simulink model "pmsm_drive_st"  (R2014a)
settings: Solver=ode3  SolverMode=SingleTasking  StartTime=0.0  StopTime=1  FixedStep=Ts  RelTol=1e-4
PreLoadFcn:
  | Ts=1e-5;
InitFcn:
  | Ts=1e-5;
StartFcn:
  | tic;
StopFcn:
  | toc;
undefined symbols (not defined in the file or in its folder): Acid, DiscIntNeverNeededParam, Lead
libraries: powerlib x10, electricdrivelib x1
Description:
  | Copyright 2008 The MathWorks(TM), Inc.
settings Model: ExtModeTrigMode=oneshot  ExtModeArmWhenConnect=off  ExtModeAutoUpdateStatusClock=off  Creator=patrice  LastModifiedBy=cosorio
settings DataIOCC: ExternalInput=[]  LimitDataPoints=off  SignalLoggingSaveFormat=ModelDataLogs  SaveOutput=off  SaveTime=off  SignalLoggingName=sigsOut
settings OptimizationCC: BlockReduction=off  BooleanDataType=off  ExpressionDepthLimit=2147483647  InitFltsAndDblsToZero=on  EfficientMapNaN2IntZero=off  OptimizeModelRefInitCode=on  LifeSpan=1
settings DebuggingCC: UnderspecifiedInitializationDetection=Classic  CheckExecutionContextPreStartOutputMsg=on  CheckExecutionContextRuntimeOutputMsg=on  SignalResolutionControl=TryResolveAllWithWarning  SolverPrmCheckMsg=none  MultiTaskDSMMsg=warning  MultiTaskCondExecSysMsg=none  SigSpecEnsureSampleTimeMsg=none  FcnCallInpInsideContextMsg=UseLocalSettings  StateNameClashWarn=warning
settings HardwareCC: TargetLongLongMode=on  TargetIntDivRoundTo=Zero  TargetEndianess=LittleEndian  TargetHWDeviceType=MATLAB Host  ProdEqTarget=off
settings RTWCC: SystemTargetFile=ert.tlc  TemplateMakefile=ert_default_tmf  Description=Embedded Coder  GenerateReport=on  ProcessScript=ert_make_rtw_hook  IncludeHyperlinkInReport=on  LaunchReport=on  IncludeERTFirstTime=on  GenerateTraceInfo=on  GenerateTraceReport=on  GenerateTraceReportSl=on  GenerateTraceReportSf=on  GenerateTraceReportEml=on  GenerateWebview=on  GenerateCodeMetricsReport=on
settings CodeAppCC: IgnoreCustomStorageClasses=off
settings ERTTargetCC: ParMdlRefBuildCompliant=on  CompOptLevelCompliant=on  ConcurrentExecutionCompliant=on  ERTFirstTimeCompliant=on  ModelStepFunctionPrototypeControlCompliant=on  CPPClassGenCompliant=on  InlinedParameterPlacement=Hierarchical  ERTCustomFileTemplate=example_file_process.tlc
settings SimscapeCC: ExplicitSolverDiagnosticOptions=none

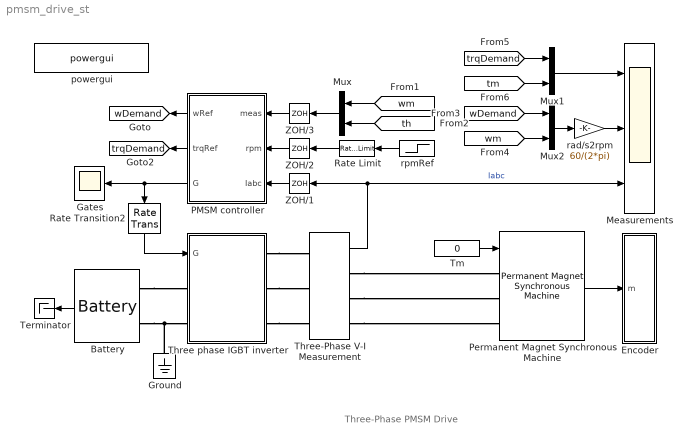
== system pmsm_drive_st ==
  note: Three-Phase PMSM Drive
  Battery : electricdrivelib/Extra Sources/Battery  BatType=Lead-Acid  ShowDetailedParameters=off  NomV=500  NomQ=1200  SOC=80  PresetModel=off  MaxQ=1250  FullV=517  Dis_rate=240  R=0.0041667  Normal_OP=372.3333  expZone="[512           4]"  Dis_Char=off  current=[10 30]  Units=Ampere-hour  Batt_Tr=1
  Encoder : Subsystem
  Gates : Scope
      settings: YMin=-0.2  YMax=1.2  MaxDataPoints=50000
  Ground : powerlib/Elements/Ground  LConnTagsString=a
  Measurements : Scope  NumInputPorts=3
      settings: YMin=-100~0~-2200  YMax=600~250~2200  SaveName=ScopeData4  MaxDataPoints=50000
  Mux : Mux  Inputs=2
  Mux1 : Mux  Inputs=2
  Mux2 : Mux  Inputs=2
  PMSM controller : Subsystem  TreatAsAtomicUnit=on  SystemSampleTime=1e-4
  Permanent Magnet Synchronous Machine : powerlib/Machines/Permanent Magnet Synchronous Machine  NbPhases=3  FluxDistribution=Sinusoidal  RotorType=Salient-pole  MechanicalLoad=Torque Tm  PresetModel=No  ShowDetailedParameters=on  MeasurementBus=off  Resistance=0.013  Inductance=8.5e-3  dqInductances=[0.0002, 0.0001995]  La=0.000835  MachineConstant=Flux linkage established by magnets (V.s)  Flux=0.03  VoltageCst=32.6484  TorqueCst=0.27  Flat=0  Mechanical=[10, 0, 6]  PolePairs=4  InitialConditions=[0,0, 166,-166]  InitialConditions5ph=[0 0 0 0 0 0]  TsPowergui=0  TsBlock=-1  RefAngle=90 degrees behind phase A axis (modified Park)
      settings: AttributesFormatString=\n
  Rate Limit : RateLimiter  RisingSlewLimit=400  FallingSlewLimit=-400  SampleTimeMode=inherited
  Rate Transition2 : RateTransition
  Terminator : Terminator
  Three phase IGBT inverter : Subsystem
  Three-Phase V-I Measurement : powerlib/Measurements/Three-Phase V-I Measurement  VoltageMeasurement=no  SetLabelV=off  LabelV=Vabc  Vpu=off  VpuLL=off  CurrentMeasurement=yes  SetLabelI=off  LabelI=Iabc  Ipu=off  Pbase=100e6  Vbase=500e3  OutputType=Complex  PhasorSimulation=off  PSBequivalent=0
  Tm : Constant  Value=0  SampleTime=Ts
  ZOH/1 : ZeroOrderHold  SampleTime=1e-4
  ZOH/2 : ZeroOrderHold  SampleTime=1e-4
  ZOH/3 : ZeroOrderHold  SampleTime=1e-4
  powergui : powerlib/powergui  SimulationMode=Discrete  SolverType=Tustin  SampleTime=Ts  frequency=60  SPID=off  DisableSnubberDevices=off  DisableRonSwitches=off  DisableVfSwitches=off  SwTol=0  Interpol=off  DisplayEquations=off  Ts=0  methode=off  frequencyindice=0  Pbase=100e6  ErrMax=1e-4  Iterations=50  UnitsV=kV  UnitsW=MW  FunctionMessages=off  echomessages=off  HookPort=off  EnableUseOfTLC=off  x0status=blocks  RestoreLinks=warning  ResistiveCurrentMeasurement=off  Frange=[0:2:500]  Ylog=off  Xlog=on  ShowGrid=off  save=off  variable=ZData  structure=Vmod  ZoomFFT=on  StartTime=2.4  cycles=10  DisplayStyle=1  fundamental=100  FreqAxis=on  MaxFrequency=6500  frequencyindicesteady=1  RmsSteady=1  display=off
  rad/s2rpm : Gain  Gain=60/(2*pi)
  rpmRef : Step  Time=0.1  After=200  SampleTime=1e-4
  tag scope: trqDemand=global, wDemand=global
  wires:
  rpmRef/1 -> Rate Limit/1
  ZOH/1/1 -> PMSM controller/3(Iabc)
  ZOH/2/1 -> PMSM controller/2(rpm)
  ZOH/3/1 -> PMSM controller/1(meas)
  [th] -> Mux/2
  [wm] -> Mux/1
  Mux/1 -> ZOH/3/1
  rad/s2rpm/1 -> Measurements/2
  Mux2/1 -> rad/s2rpm/1
  [wm] -> Mux2/2
  [wDemand] -> Mux2/1
  Mux1/1 -> Measurements/1
  [tm] -> Mux1/2
  [trqDemand] -> Mux1/1
  Battery/1 -> Terminator/1
  PMSM controller/3(G) -> Rate Transition2/1, Gates/1
  Rate Transition2/1 -> Three phase IGBT inverter/1(G)
  Permanent Magnet Synchronous Machine/1 -> Encoder/1(m)
  Tm/1 -> Permanent Magnet Synchronous Machine/1
  Rate Limit/1 -> ZOH/2/1
  Three-Phase V-I Measurement/1 -> Measurements/3, ZOH/1/1  "Iabc"
  PMSM controller/1(wRef) -> [wDemand]
  PMSM controller/2(trqRef) -> [trqDemand]
  connections:
  Battery/LConn2 -- Ground/LConn1 -- Three phase IGBT inverter/LConn2
  Battery/LConn1 -- Three phase IGBT inverter/LConn1
  Three-Phase V-I Measurement/RConn1 -- Permanent Magnet Synchronous Machine/LConn1
  Three-Phase V-I Measurement/RConn2 -- Permanent Magnet Synchronous Machine/LConn2
  Three-Phase V-I Measurement/RConn3 -- Permanent Magnet Synchronous Machine/LConn3
  Three phase IGBT inverter/RConn1 -- Three-Phase V-I Measurement/LConn1
  Three phase IGBT inverter/RConn2 -- Three-Phase V-I Measurement/LConn2
  Three phase IGBT inverter/RConn3 -- Three-Phase V-I Measurement/LConn3

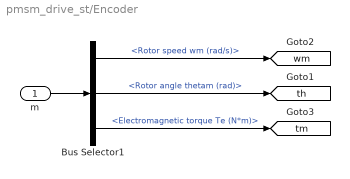
== system pmsm_drive_st/Encoder ==
  m : Inport
  Bus Selector1 : BusSelector  OutputSignals=Rotor speed wm (rad/s),Rotor angle thetam (rad),Electromagnetic torque Te (N*m)
  tag scope: th=global, tm=global, wm=global
  wires:
  Bus Selector1/1 -> [wm]  "<Rotor speed wm (rad/s)>"
  Bus Selector1/3 -> [tm]  "<Electromagnetic torque Te (N*m)>"
  m/1 -> Bus Selector1/1
  Bus Selector1/2 -> [th]  "<Rotor angle thetam (rad)>"

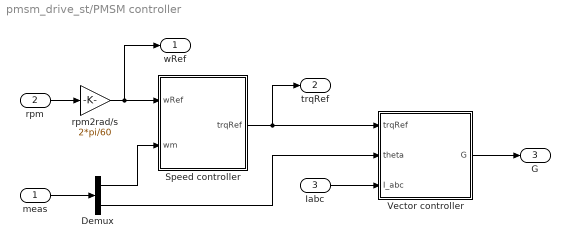
== system pmsm_drive_st/PMSM controller ==
  meas : Inport  OutDataTypeStr=double  PortDimensions=2  SampleTime=1e-4
  rpm : Inport  Port=2  OutDataTypeStr=double  PortDimensions=1  SampleTime=1e-4
  Iabc : Inport  Port=3  OutDataTypeStr=double  PortDimensions=3  SampleTime=1e-4
  Demux : Demux  Outputs=2
  Speed controller : Subsystem  mask(P+I motor speed controller){Kp=10000, Ki=10000, trqMax=500, ts=1e-4}
      mask prompts: Kp "Proportional gain (Nm/(rad/s))"; Ki "Integral gain (Nm/rad)"; trqMax "Maximum torque demand"; ts "Sample time"
      mask help: Inputs wRef and wMeas are the demanded rotor speed and measured rotor speed in rad/s. The controller output is a torque demand in Nm.
  Vector controller : Subsystem  mask(Vector controller){Np=6, lambda=0.03, h=1}
      mask prompts: Np "Number of pole pairs, p"; lambda "Flux linkage from rotor permanent magnet"; h "Current hysteresis (A)"
  rpm2rad/s : Gain  Gain=2*pi/60
  wRef : Outport  OutDataTypeStr=double  PortDimensions=1  SampleTime=1e-4
  trqRef : Outport  Port=2  OutDataTypeStr=double  PortDimensions=1  SampleTime=1e-4
  G : Outport  Port=3  OutDataTypeStr=double  PortDimensions=6  SampleTime=1e-4
  wires:
  Vector controller/1(G) -> G/1
  Speed controller/1(trqRef) -> trqRef/1, Vector controller/1(trqRef)
  Iabc/1 -> Vector controller/3(I_abc)
  rpm/1 -> rpm2rad/s/1
  rpm2rad/s/1 -> Speed controller/1(wRef), wRef/1
  meas/1 -> Demux/1
  Demux/1 -> Speed controller/2(wm)
  Demux/2 -> Vector controller/2(theta)

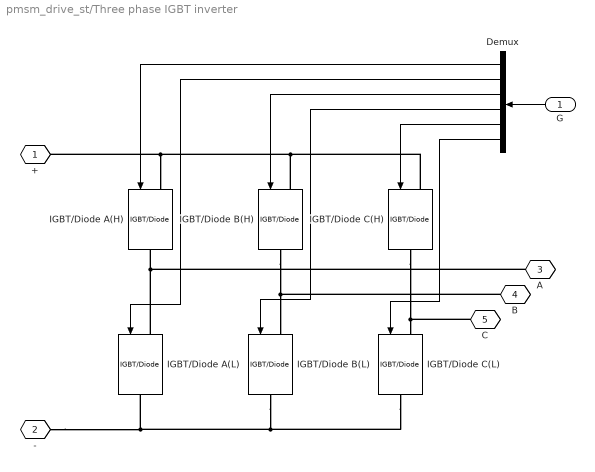
== system pmsm_drive_st/Three phase IGBT inverter ==
  G : Inport
  Demux : Demux  Outputs=6
  IGBT/Diode A(H) : powerlib/Power Electronics/IGBT//Diode  Ron=0.001  Rs=1e5  Cs=inf  Measurements=off
  IGBT/Diode A(L) : powerlib/Power Electronics/IGBT//Diode  Ron=0.001  Rs=1e5  Cs=inf  Measurements=off
  IGBT/Diode B(H) : powerlib/Power Electronics/IGBT//Diode  Ron=0.001  Rs=1e5  Cs=inf  Measurements=off
  IGBT/Diode B(L) : powerlib/Power Electronics/IGBT//Diode  Ron=0.001  Rs=1e5  Cs=inf  Measurements=off
  IGBT/Diode C(H) : powerlib/Power Electronics/IGBT//Diode  Ron=0.001  Rs=1e5  Cs=inf  Measurements=off
  IGBT/Diode C(L) : powerlib/Power Electronics/IGBT//Diode  Ron=0.001  Rs=1e5  Cs=inf  Measurements=off
  + : PMIOPort  Tag=PMCPort  Port=1  Side=Left
  - : PMIOPort  Tag=PMCPort  Port=2  Side=Left
  A : PMIOPort  Tag=PMCPort  Port=3  Side=Right
  B : PMIOPort  Tag=PMCPort  Port=4  Side=Right
  C : PMIOPort  Tag=PMCPort  Port=5  Side=Right
  wires:
  Demux/3 -> IGBT/Diode B(H)/1
  Demux/4 -> IGBT/Diode B(L)/1
  Demux/1 -> IGBT/Diode A(H)/1
  Demux/2 -> IGBT/Diode A(L)/1
  Demux/5 -> IGBT/Diode C(H)/1
  Demux/6 -> IGBT/Diode C(L)/1
  G/1 -> Demux/1
  connections:
  IGBT/Diode B(H)/RConn1 -- B/RConn1 -- IGBT/Diode B(L)/LConn1
  IGBT/Diode B(H)/LConn1 -- IGBT/Diode C(H)/LConn1 -- +/RConn1 -- IGBT/Diode A(H)/LConn1
  IGBT/Diode A(L)/LConn1 -- IGBT/Diode A(H)/RConn1 -- A/RConn1
  IGBT/Diode B(L)/RConn1 -- IGBT/Diode A(L)/RConn1 -- -/RConn1 -- IGBT/Diode C(L)/RConn1
  IGBT/Diode C(H)/RConn1 -- C/RConn1 -- IGBT/Diode C(L)/LConn1

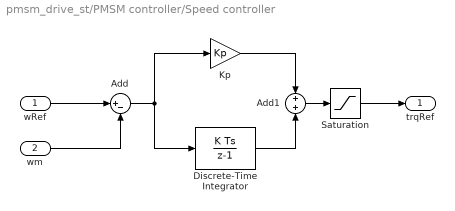
== system pmsm_drive_st/PMSM controller/Speed controller ==
  wRef : Inport
  wm : Inport  Port=2
  Add : Sum  Inputs=|+-
  Add1 : Sum
  Discrete-Time Integrator : DiscreteIntegrator  gainval=Ki  SampleTime=ts  LimitOutput=on  UpperSaturationLimit=trqMax  LowerSaturationLimit=-trqMax  ICPrevOutput=DiscIntNeverNeededParam  ICPrevScaledInput=DiscIntNeverNeededParam
  Kp : Gain  Gain=Kp
  Saturation : Saturate  UpperLimit=trqMax  LowerLimit=-trqMax
  trqRef : Outport
  wires:
  wRef/1 -> Add/1
  Add1/1 -> Saturation/1
  Kp/1 -> Add1/1
  Discrete-Time Integrator/1 -> Add1/2
  wm/1 -> Add/2
  Saturation/1 -> trqRef/1
  Add/1 -> Kp/1, Discrete-Time Integrator/1

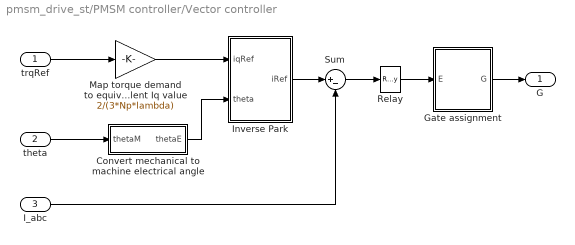
== system pmsm_drive_st/PMSM controller/Vector controller ==
  trqRef : Inport
  theta : Inport  Port=2
  I_abc : Inport  Port=3
  Convert mechanical to machine electrical angle : Subsystem
  Gate assignment : Subsystem
  Inverse Park : Subsystem
  Map torque demand to equivalent Iq value : Gain  Gain=2/(3*Np*lambda)  SaturateOnIntegerOverflow=on  OutDataTypeStr=Inherit: Same as input  ParamDataTypeStr=Inherit: Same as input
  Relay : Relay  OnSwitchValue=h/2  OffSwitchValue=-h/2
  Sum : Sum  Inputs=|+-  SaturateOnIntegerOverflow=on  InputSameDT=on  OutDataTypeStr=Inherit: Same as first input
  G : Outport
  wires:
  Convert mechanical to machine electrical angle/1(thetaE) -> Inverse Park/2(theta)
  theta/1 -> Convert mechanical to machine electrical angle/1(thetaM)
  Map torque demand to equivalent Iq value/1 -> Inverse Park/1(iqRef)
  I_abc/1 -> Sum/2
  trqRef/1 -> Map torque demand to equivalent Iq value/1
  Inverse Park/1(iRef) -> Sum/1
  Sum/1 -> Relay/1
  Relay/1 -> Gate assignment/1(E)
  Gate assignment/1(G) -> G/1

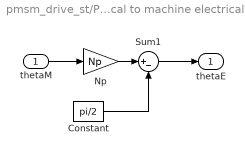
== system pmsm_drive_st/PMSM controller/Vector controller/Convert mechanical to machine electrical angle ==
  thetaM : Inport
  Constant : Constant  Value=pi/2
  Np : Gain  Gain=Np  SaturateOnIntegerOverflow=on  OutDataTypeStr=Inherit: Same as input  ParamDataTypeStr=Inherit: Same as input
  Sum1 : Sum  Inputs=|+-
  thetaE : Outport
  wires:
  Constant/1 -> Sum1/2
  thetaM/1 -> Np/1
  Np/1 -> Sum1/1
  Sum1/1 -> thetaE/1

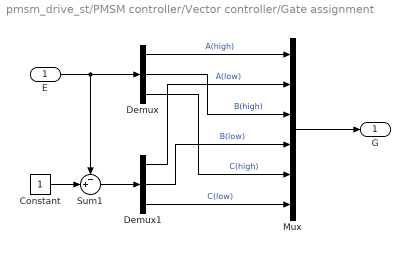
== system pmsm_drive_st/PMSM controller/Vector controller/Gate assignment ==
  E : Inport
  Constant : Constant
  Demux : Demux  Outputs=3
  Demux1 : Demux  Outputs=3
  Mux : Mux  Inputs=6
  Sum1 : Sum  Inputs=-+|  SaturateOnIntegerOverflow=on  InputSameDT=on  OutDataTypeStr=Inherit: Same as first input
  G : Outport
  wires:
  Demux/3 -> Mux/5  "C(high)"
  Demux1/3 -> Mux/6  "C(low)"
  Mux/1 -> G/1
  Sum1/1 -> Demux1/1
  E/1 -> Sum1/1, Demux/1
  Constant/1 -> Sum1/2
  Demux/1 -> Mux/1  "A(high)"
  Demux/2 -> Mux/3  "B(high)"
  Demux1/2 -> Mux/4  "B(low)"
  Demux1/1 -> Mux/2  "A(low)"

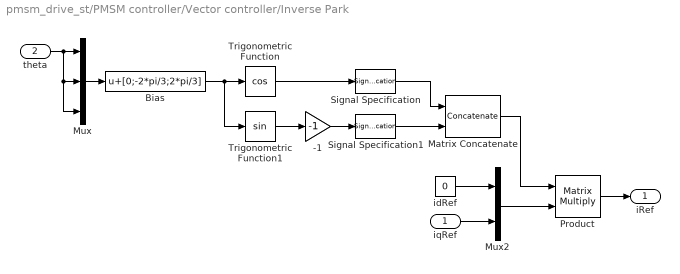
== system pmsm_drive_st/PMSM controller/Vector controller/Inverse Park ==
  iqRef : Inport
  theta : Inport  Port=2
  -1 : Gain  Gain=-1  SaturateOnIntegerOverflow=on  OutDataTypeStr=Inherit: Same as input  ParamDataTypeStr=Inherit: Same as input
  Bias : Bias  Bias=[0;-2*pi/3;2*pi/3]
  Matrix Concatenate : Concatenate  Mode=Multidimensional array  ConcatenateDimension=2
  Mux : Mux  Inputs=3
  Mux2 : Mux  Inputs=2
  Product : Product  Multiplication=Matrix(*)  RndMeth=Zero
  Signal Specification : SignalSpecification  Dimensions=[3 1]
  Signal Specification1 : SignalSpecification  Dimensions=[3 1]
  Trigonometric Function : Trigonometry  Operator=cos
  Trigonometric Function1 : Trigonometry
  idRef : Constant  Value=0
  iRef : Outport  InitialOutput=0
  wires:
  Mux/1 -> Bias/1
  Matrix Concatenate/1 -> Product/1
  Mux2/1 -> Product/2
  iqRef/1 -> Mux2/2
  idRef/1 -> Mux2/1
  Signal Specification/1 -> Matrix Concatenate/1
  Signal Specification1/1 -> Matrix Concatenate/2
  Trigonometric Function1/1 -> -1/1
  Bias/1 -> Trigonometric Function/1, Trigonometric Function1/1
  theta/1 -> Mux/3, Mux/2, Mux/1
  Product/1 -> iRef/1
  Trigonometric Function/1 -> Signal Specification/1
  -1/1 -> Signal Specification1/1
